simulink model "minseg_M2V3_2017a"  (R2017a)
settings: Solver=FixedStepDiscrete  StartTime=0.0  StopTime=inf  FixedStep=mdl_T_sample  RelTol=1e-3
undefined symbols (not defined in the file or in its folder): ctrl_lqr_K2, ctrl_motorDriver_v_ff_cmd_v_val, ctrl_motorDriver_v_ff_cmd_v_val_norm_dx_max, ctrl_motorDriver_v_ff_cmd_v_val_norm_dx_min, ctrl_motorDriver_v_output_max, ctrl_motorDriver_v_output_min, ctrl_motorDriver_v_pid_cmd_thetaDot_val, ctrl_motorDriver_v_pid_cmd_thetaDot_val_norm_dx_max, ctrl_motorDriver_v_pid_cmd_thetaDot_val_norm_dx_min, ctrl_motorDriver_v_pid_int_maxVal, ctrl_motorDriver_v_pid_int_minVal, ctrl_motorDriver_v_pid_k_d, ctrl_motorDriver_v_pid_k_i, ctrl_motorDriver_v_pid_k_p, ctrl_motorDriver_v_rts_ss_k_A, ctrl_motorDriver_v_rts_ss_k_B, ctrl_motorDriver_v_rts_ss_k_C, ctrl_motorDriver_v_rts_ss_k_D, ctrl_motorDriver_v_rts_ss_stateIC, ctrl_motorDriver_v_sfr_cmd_p_x_f, ctrl_motorDriver_v_sfr_cmd_p_x_mag, ctrl_motorDriver_v_sfr_cmd_p_y_f, ctrl_motorDriver_v_sfr_cmd_p_y_mag, ctrl_motorDriver_v_sfr_K, ctrl_motorDriver_v_sfr_K_plant, ctrl_motorDriver_v_sfr_K_rts, ctrl_motorDriver_v_T_cmd, ctrl_motorDriver_v_T_init, DiscIntNeverNeededParam, gyro_bias, io_srl_read_rateTransition_initialCondition, k_intmax_uint8, mdl_T_sample, mtr_encoder_filter_z_ss_A, mtr_encoder_filter_z_ss_B, mtr_encoder_filter_z_ss_C, mtr_encoder_filter_z_ss_D, plant, plant_accel_k_digital2analog, plant_body_l_c, plant_body_l_w, plant_gyro_encoder_filter_z_den, plant_gyro_encoder_filter_z_num, plant_gyro_filter_z_den, plant_gyro_filter_z_num, plant_gyro_k_digital2analog, plant_linear_ss_stateIC, plant_linear_ss_t_A, plant_linear_ss_t_B, plant_linear_ss_t_C, plant_linear_ss_t_D, plant_mtr_encoder_count2wheelRad, plant_mtr_encoder_filter_z_den, plant_mtr_encoder_filter_z_num, plant_pSupply_v, plant_supply_v, plant_T_init, plant_wheel_r
undefined symbols (not defined in the file): ctrl_lqr_addlDyn_A_discrete, ctrl_lqr_addlDyn_B_discrete, ctrl_lqr_addlDyn_C_discrete, ctrl_lqr_addlDyn_D_discrete, ctrl_lqr_addlDyn_k_antiWindup, ctrl_lqr_addlDyn_stateIC, plant_gyro_bias_movingAverage_n_pts, plant_linear_A_continuous, plant_linear_B_continuous, plant_linear_C_continuous, plant_linear_D_continuous, plant_linear_stateIC
libraries: svdutilitieslib x135, simulink x57, arduinolib x15, MinSegLibrary_M2V3 x3, dspindex x3, RASPlib x2
(part 6 of 6)

== system minseg_M2V3_2017a/Plant/Hardware/Calculations/Linear Position (p)/Wheel/Middle-Connected ==
  p.center.x : Inport
  p.center.y : Inport  Port=2
  p.center.z : Inport  Port=3
  body.angularPosition.y (yaw) : Inport  Port=4
  Add1 : Sum
  Add2 : Sum
  Bus Creator : BusCreator  Inputs=2
  Bus Creator1 : BusCreator  Inputs=2
  Bus Creator2 : BusCreator  Inputs=2
  Discrete Derivative [Average] : simulink/Discrete/Discrete Derivative  gainval=1.0  ICPrevScaledInput=0  OutMin=[]  OutMax=[]  OutDataType=fixdt(1, 16)  OutScaling=2^-10  DoSatur=off
      settings: AttributesFormatString=initialCondition = %<ICPrevScaledInput>
  Discrete Derivative [Left-Connected] : simulink/Discrete/Discrete Derivative  gainval=1.0  ICPrevScaledInput=0  OutMin=[]  OutMax=[]  OutDataType=fixdt(1, 16)  OutScaling=2^-10  DoSatur=off
      settings: AttributesFormatString=initialCondition = %<ICPrevScaledInput>
  Discrete Derivative [Middle-Connected] : simulink/Discrete/Discrete Derivative  gainval=1.0  ICPrevScaledInput=0  OutMin=[]  OutMax=[]  OutDataType=fixdt(1, 16)  OutScaling=2^-10  DoSatur=off
      settings: AttributesFormatString=initialCondition = %<ICPrevScaledInput>
  Gain3 : Gain  Gain=+ plant_body_l_w / 2
      settings: AttributesFormatString=%<Gain>
  Gain4 : Gain  Gain=- plant_body_l_w / 2
      settings: AttributesFormatString=%<Gain>
  Trigonometric Function : Trigonometry
  Trigonometric Function1 : Trigonometry  Operator=cos
  x : Outport
  y : Outport  Port=2
  z : Outport  Port=3
  wires:
  Discrete Derivative [Average]/1 -> Bus Creator2/2  "velocity [m/s]"
  Discrete Derivative [Middle-Connected]/1 -> Bus Creator1/2  "velocity [m/s]"
  Discrete Derivative [Left-Connected]/1 -> Bus Creator/2  "velocity [m/s]"
  Bus Creator1/1 -> y/1
  Bus Creator/1 -> x/1
  p.center.z/1 -> Bus Creator2/1, Discrete Derivative [Average]/1  "position [m]"
  Bus Creator2/1 -> z/1
  Add2/1 -> Discrete Derivative [Middle-Connected]/1, Bus Creator1/1  "position [m]"
  Add1/1 -> Bus Creator/1, Discrete Derivative [Left-Connected]/1  "position [m]"
  [yaw] -> Trigonometric Function/1
  Trigonometric Function/1 -> Gain3/1
  p.center.x/1 -> Add1/1
  Trigonometric Function1/1 -> Gain4/1
  p.center.y/1 -> Add2/1
  body.angularPosition.y (yaw)/1 -> [yaw]
  [yaw] -> Trigonometric Function1/1
  Gain3/1 -> Add1/2
  Gain4/1 -> Add2/2

== system minseg_M2V3_2017a/Plant/Hardware/Digital to Analog Conversion/Gyroscope/x/Moving Average ==
  u : Inport
  Enable : EnablePort
  Gain : Gain  Gain=ones(1,N) / N  Multiplication=Matrix(K*u)
      settings: AttributesFormatString=%<Gain>
  Mux : Mux  Inputs=2
  Unit Delay : UnitDelay  InitialCondition=zeros(N-1,1)  SampleTime=-1
  Variable Selector : dspindex/Variable Selector  NumInputs=1  rowsOrCols=Rows  IdxMode=Fixed  Elements=[ 1 : (N-1) ]  ZerOneIdxMode=One-based  errmode=Clip Index  FillMode=on  FillValues=0
  u.avg : Outport
  wires:
  Mux/1 -> Variable Selector/1, Gain/1
  Variable Selector/1 -> Unit Delay/1
  Gain/1 -> u.avg/1
  Unit Delay/1 -> Mux/2
  u/1 -> Mux/1

== system minseg_M2V3_2017a/Plant/Hardware/Digital to Analog Conversion/Gyroscope/y/Moving Average ==
  u : Inport
  Enable : EnablePort
  Gain : Gain  Gain=ones(1,N) / N  Multiplication=Matrix(K*u)
      settings: AttributesFormatString=%<Gain>
  Mux : Mux  Inputs=2
  Unit Delay : UnitDelay  InitialCondition=zeros(N-1,1)  SampleTime=-1
  Variable Selector : dspindex/Variable Selector  NumInputs=1  rowsOrCols=Rows  IdxMode=Fixed  Elements=[ 1 : (N-1) ]  ZerOneIdxMode=One-based  errmode=Clip Index  FillMode=on  FillValues=0
  u.avg : Outport
  wires:
  Mux/1 -> Variable Selector/1, Gain/1
  Variable Selector/1 -> Unit Delay/1
  Gain/1 -> u.avg/1
  Unit Delay/1 -> Mux/2
  u/1 -> Mux/1

== system minseg_M2V3_2017a/Plant/Hardware/Digital to Analog Conversion/Gyroscope/z/Moving Average ==
  u : Inport
  Enable : EnablePort
  Gain : Gain  Gain=ones(1,N) / N  Multiplication=Matrix(K*u)
      settings: AttributesFormatString=%<Gain>
  Mux : Mux  Inputs=2
  Unit Delay : UnitDelay  InitialCondition=zeros(N-1,1)  SampleTime=-1
  Variable Selector : dspindex/Variable Selector  NumInputs=1  rowsOrCols=Rows  IdxMode=Fixed  Elements=[ 1 : (N-1) ]  ZerOneIdxMode=One-based  errmode=Clip Index  FillMode=on  FillValues=0
  u.avg : Outport
  wires:
  Mux/1 -> Variable Selector/1, Gain/1
  Variable Selector/1 -> Unit Delay/1
  Gain/1 -> u.avg/1
  Unit Delay/1 -> Mux/2
  u/1 -> Mux/1

== system minseg_M2V3_2017a/Plant/Hardware-Equivalent Linear Dynamics/Calculation/Linear Position (p)/Wheel/Center ==
  wheel.angularVelocity.global : Inport
  body.angularPosition.y (yaw) : Inport  Port=2
  Add1 : Sum
  Bus Creator : BusCreator  Inputs=2
  Bus Creator1 : BusCreator  Inputs=2
  Bus Creator2 : BusCreator  Inputs=2
  Constant : Constant  Value=0  SampleTime=mdl_T_sample
  Constant1 : Constant  Value=plant.wheel.r  SampleTime=mdl_T_sample
      settings: AttributesFormatString=%<Value>
  Discrete-Time Integrator (X) : DiscreteIntegrator  InitialConditionSetting=State (most efficient)  SampleTime=-1  ICPrevOutput=DiscIntNeverNeededParam  ICPrevScaledInput=DiscIntNeverNeededParam
      settings: AttributesFormatString=initialCondition = %<InitialCondition>
  Discrete-Time Integrator (Y) : DiscreteIntegrator  InitialConditionSetting=State (most efficient)  SampleTime=-1  ICPrevOutput=DiscIntNeverNeededParam  ICPrevScaledInput=DiscIntNeverNeededParam
      settings: AttributesFormatString=initialCondition = %<InitialCondition>
  Discrete-Time Integrator (Z) : DiscreteIntegrator  InitialConditionSetting=State (most efficient)  SampleTime=-1  ICPrevOutput=DiscIntNeverNeededParam  ICPrevScaledInput=DiscIntNeverNeededParam
      settings: AttributesFormatString=initialCondition = %<InitialCondition>
  Gain3 : Gain  Gain=plant_wheel_r
      settings: AttributesFormatString=%<Gain>
  Gain4 : Gain  Gain=plant_wheel_r
      settings: AttributesFormatString=%<Gain>
  Product : Product
  Product1 : Product
  Trigonometric Function : Trigonometry  Operator=cos
  Trigonometric Function1 : Trigonometry
  x : Outport
  y : Outport  Port=2
  z : Outport  Port=3
  wires:
  Bus Creator2/1 -> z/1
  Bus Creator/1 -> x/1
  Bus Creator1/1 -> y/1
  Product/1 -> Discrete-Time Integrator (X)/1, Bus Creator/2  "velocity [m/s]"
  Product1/1 -> Discrete-Time Integrator (Y)/1, Bus Creator1/2  "velocity  [m/s]"
  Constant/1 -> Discrete-Time Integrator (Z)/1, Bus Creator2/2  "velocity [m/s]"
  Discrete-Time Integrator (X)/1 -> Bus Creator/1  "position [m]"
  Discrete-Time Integrator (Y)/1 -> Bus Creator1/1  "position [m]"
  Add1/1 -> Bus Creator2/1  "position [m]"
  wheel.angularVelocity.global/1 -> [theta_dot]
  Gain3/1 -> Product/1
  Trigonometric Function/1 -> Product/2
  body.angularPosition.y (yaw)/1 -> [yaw]
  Trigonometric Function1/1 -> Product1/2
  Gain4/1 -> Product1/1
  [yaw] -> Trigonometric Function/1
  [theta_dot] -> Gain3/1
  [theta_dot] -> Gain4/1
  [yaw] -> Trigonometric Function1/1
  Discrete-Time Integrator (Z)/1 -> Add1/2
  Constant1/1 -> Add1/1

== system minseg_M2V3_2017a/Plant/Hardware-Equivalent Linear Dynamics/Calculation/Linear Position (p)/Wheel/Left-Connected ==
  p.center.x : Inport
  p.center.y : Inport  Port=2
  p.center.z : Inport  Port=3
  body.angularPosition.y (yaw) : Inport  Port=4
  Add1 : Sum
  Add2 : Sum
  Bus Creator : BusCreator  Inputs=2
  Bus Creator1 : BusCreator  Inputs=2
  Bus Creator2 : BusCreator  Inputs=2
  Discrete Derivative (X) : simulink/Discrete/Discrete Derivative  gainval=1.0  ICPrevScaledInput=0  OutMin=[]  OutMax=[]  OutDataType=fixdt(1, 16)  OutScaling=2^-10  DoSatur=off
      settings: AttributesFormatString=initialCondition = %<ICPrevScaledInput>
  Discrete Derivative (Y) : simulink/Discrete/Discrete Derivative  gainval=1.0  ICPrevScaledInput=0  OutMin=[]  OutMax=[]  OutDataType=fixdt(1, 16)  OutScaling=2^-10  DoSatur=off
      settings: AttributesFormatString=initialCondition = %<ICPrevScaledInput>
  Discrete Derivative (Z) : simulink/Discrete/Discrete Derivative  gainval=1.0  ICPrevScaledInput=0  OutMin=[]  OutMax=[]  OutDataType=fixdt(1, 16)  OutScaling=2^-10  DoSatur=off
      settings: AttributesFormatString=initialCondition = %<ICPrevScaledInput>
  Gain3 : Gain  Gain=- plant_body_l_w / 2
      settings: AttributesFormatString=%<Gain>
  Gain4 : Gain  Gain=+ plant_body_l_w / 2
      settings: AttributesFormatString=%<Gain>
  Trigonometric Function : Trigonometry
  Trigonometric Function1 : Trigonometry  Operator=cos
  x : Outport
  y : Outport  Port=2
  z : Outport  Port=3
  wires:
  Gain4/1 -> Add2/2
  Gain3/1 -> Add1/2
  [yaw] -> Trigonometric Function1/1
  body.angularPosition.y (yaw)/1 -> [yaw]
  p.center.y/1 -> Add2/1
  Trigonometric Function1/1 -> Gain4/1
  p.center.x/1 -> Add1/1
  Trigonometric Function/1 -> Gain3/1
  [yaw] -> Trigonometric Function/1
  Add1/1 -> Discrete Derivative (X)/1, Bus Creator/1  "position [m]"
  Add2/1 -> Discrete Derivative (Y)/1, Bus Creator1/1  "position [m]"
  Bus Creator2/1 -> z/1
  p.center.z/1 -> Discrete Derivative (Z)/1, Bus Creator2/1  "position [m]"
  Bus Creator/1 -> x/1
  Bus Creator1/1 -> y/1
  Discrete Derivative (X)/1 -> Bus Creator/2  "velocity [m/s]"
  Discrete Derivative (Y)/1 -> Bus Creator1/2  "velocity [m/s]"
  Discrete Derivative (Z)/1 -> Bus Creator2/2  "velocity [m/s]"

== system minseg_M2V3_2017a/Plant/Hardware-Equivalent Linear Dynamics/Calculation/Linear Position (p)/Wheel/Middle-Connected ==
  p.center.x : Inport
  p.center.y : Inport  Port=2
  p.center.z : Inport  Port=3
  body.angularPosition.y (yaw) : Inport  Port=4
  Add1 : Sum
  Add2 : Sum
  Bus Creator : BusCreator  Inputs=2
  Bus Creator1 : BusCreator  Inputs=2
  Bus Creator2 : BusCreator  Inputs=2
  Discrete Derivative (X) : simulink/Discrete/Discrete Derivative  gainval=1.0  ICPrevScaledInput=0  OutMin=[]  OutMax=[]  OutDataType=fixdt(1, 16)  OutScaling=2^-10  DoSatur=off
      settings: AttributesFormatString=initialCondition = %<ICPrevScaledInput>
  Discrete Derivative (Y) : simulink/Discrete/Discrete Derivative  gainval=1.0  ICPrevScaledInput=0  OutMin=[]  OutMax=[]  OutDataType=fixdt(1, 16)  OutScaling=2^-10  DoSatur=off
      settings: AttributesFormatString=initialCondition = %<ICPrevScaledInput>
  Discrete Derivative (Z) : simulink/Discrete/Discrete Derivative  gainval=1.0  ICPrevScaledInput=0  OutMin=[]  OutMax=[]  OutDataType=fixdt(1, 16)  OutScaling=2^-10  DoSatur=off
      settings: AttributesFormatString=initialCondition = %<ICPrevScaledInput>
  Gain3 : Gain  Gain=+ plant_body_l_w / 2
      settings: AttributesFormatString=%<Gain>
  Gain4 : Gain  Gain=- plant_body_l_w / 2
      settings: AttributesFormatString=%<Gain>
  Trigonometric Function : Trigonometry
  Trigonometric Function1 : Trigonometry  Operator=cos
  x : Outport
  y : Outport  Port=2
  z : Outport  Port=3
  wires:
  Discrete Derivative (Z)/1 -> Bus Creator2/2  "velocity [m/s]"
  Discrete Derivative (Y)/1 -> Bus Creator1/2  "velocity [m/s]"
  Discrete Derivative (X)/1 -> Bus Creator/2  "velocity  [m/s]"
  Bus Creator1/1 -> y/1
  Bus Creator/1 -> x/1
  p.center.z/1 -> Discrete Derivative (Z)/1, Bus Creator2/1  "position [m]"
  Bus Creator2/1 -> z/1
  Add2/1 -> Discrete Derivative (Y)/1, Bus Creator1/1  "position [m]"
  Add1/1 -> Discrete Derivative (X)/1, Bus Creator/1  "position [m]"
  [yaw] -> Trigonometric Function/1
  Trigonometric Function/1 -> Gain3/1
  p.center.x/1 -> Add1/1
  Trigonometric Function1/1 -> Gain4/1
  p.center.y/1 -> Add2/1
  body.angularPosition.y (yaw)/1 -> [yaw]
  [yaw] -> Trigonometric Function1/1
  Gain3/1 -> Add1/2
  Gain4/1 -> Add2/2

== system minseg_M2V3_2017a/User IO/Reads (From PC)/Controller/State Feedback Regulation/[x,y] to [magnitude, angle]: p/Angle ==
  u.x : Inport
  u.y : Inport  Port=2
  Trigonometric Function : Trigonometry  Operator=atan2
  "< u  " : Outport
  wires:
  u.x/1 -> Trigonometric Function/2
  u.y/1 -> Trigonometric Function/1
  Trigonometric Function/1 -> "< u  "/1

== system minseg_M2V3_2017a/User IO/Reads (From PC)/Controller/State Feedback Regulation/[x,y] to [magnitude, angle]: p/Magnitude ==
  u.x : Inport
  u.y : Inport  Port=2
  Add : Sum
  Constant1 : Constant  Value=2  SampleTime=mdl_T_sample
  Constant2 : Constant  Value=2  SampleTime=mdl_T_sample
  Math Function : Math  Operator=pow  SaturateOnIntegerOverflow=on
  Math Function1 : Math  Operator=pow  SaturateOnIntegerOverflow=on
  Sqrt : Sqrt  SaturateOnIntegerOverflow=on
  | u | : Outport
  wires:
  Math Function1/1 -> Add/2
  u.x/1 -> Math Function/1
  Math Function/1 -> Add/1
  Constant2/1 -> Math Function/2
  Constant1/1 -> Math Function1/2
  Sqrt/1 -> | u |/1
  Add/1 -> Sqrt/1
  u.y/1 -> Math Function1/1

== system minseg_M2V3_2017a/User IO/Reads (From PC)/Controller/State Feedback Regulation/[x,y] to [magnitude, angle]: p.dot/Angle ==
  u.x : Inport
  u.y : Inport  Port=2
  Trigonometric Function : Trigonometry  Operator=atan2
  "< u  " : Outport
  wires:
  Trigonometric Function/1 -> "< u  "/1
  u.y/1 -> Trigonometric Function/1
  u.x/1 -> Trigonometric Function/2

== system minseg_M2V3_2017a/User IO/Reads (From PC)/Controller/State Feedback Regulation/[x,y] to [magnitude, angle]: p.dot/Magnitude ==
  u.x : Inport
  u.y : Inport  Port=2
  Add : Sum
  Constant1 : Constant  Value=2  SampleTime=mdl_T_sample
  Constant2 : Constant  Value=2  SampleTime=mdl_T_sample
  Math Function : Math  Operator=pow  SaturateOnIntegerOverflow=on
  Math Function1 : Math  Operator=pow  SaturateOnIntegerOverflow=on
  Sqrt : Sqrt  SaturateOnIntegerOverflow=on
  | u | : Outport
  wires:
  u.y/1 -> Math Function1/1
  Add/1 -> Sqrt/1
  Sqrt/1 -> | u |/1
  Constant1/1 -> Math Function1/2
  Constant2/1 -> Math Function/2
  Math Function/1 -> Add/1
  u.x/1 -> Math Function/1
  Math Function1/1 -> Add/2

== system minseg_M2V3_2017a/User IO/Writes (To PC)/Plant: Linear Dynamics/Controller: PID/Standard/Pass Through ==
  In1 : Inport
  In2 : Inport  Port=2
  In3 : Inport  Port=3
  In4 : Inport  Port=4
  Out1 : Outport
  Out2 : Outport  Port=2
  Out3 : Outport  Port=3
  Out4 : Outport  Port=4
  wires:
  In1/1 -> Out1/1
  In2/1 -> Out2/1
  In3/1 -> Out3/1
  In4/1 -> Out4/1

== system minseg_M2V3_2017a/User IO/Writes (To PC)/Plant: Linear Dynamics/Controller: PID/Standard/Wheel ==
  wheel.angularVelocity.global : Inport
  body.angularPosition.y (yaw) : Inport  Port=2
  Bus Creator : BusCreator  Inputs=3
  Bus Creator1 : BusCreator  Inputs=3
  Bus Creator2 : BusCreator  Inputs=3
  Bus Selector3 : BusSelector  OutputSignals=x.position [m],y.position [m],z.position [m]
  Bus Selector4 : BusSelector  OutputSignals=x.position [m],y.position [m],z.position [m]
  Center : Subsystem
  Left-Connected : Subsystem
  Middle-Connected : Subsystem
  left : Outport
  middle : Outport  Port=2
  center : Outport  Port=3
  wires:
  Bus Creator/1 -> left/1
  Bus Creator1/1 -> middle/1
  body.angularPosition.y (yaw)/1 -> [yaw]
  wheel.angularVelocity.global/1 -> Center/1(wheel.angularVelocity.global)
  Left-Connected/1(x) -> Bus Creator/1  "x"
  Left-Connected/2(y) -> Bus Creator/2  "y"
  Left-Connected/3(z) -> Bus Creator/3  "z"
  Middle-Connected/1(x) -> Bus Creator1/1  "x"
  Middle-Connected/2(y) -> Bus Creator1/2  "y"
  Middle-Connected/3(z) -> Bus Creator1/3  "z"
  Center/1(x) -> Bus Creator2/1  "x"
  Center/2(y) -> Bus Creator2/2  "y"
  Center/3(z) -> Bus Creator2/3  "z"
  Bus Creator2/1 -> [p_center], center/1
  [yaw] -> Center/2(body.angularPosition.y (yaw))
  [yaw] -> Middle-Connected/4(body.angularPosition.y (yaw))
  [p_center] -> Bus Selector3/1
  Bus Selector3/1 -> Middle-Connected/1(p.center.x)  "<position [m]>"
  Bus Selector3/2 -> Middle-Connected/2(p.center.y)  "<position [m]>"
  Bus Selector3/3 -> Middle-Connected/3(p.center.z)  "<position [m]>"
  Bus Selector4/3 -> Left-Connected/3(p.center.z)  "<position [m]>"
  Bus Selector4/2 -> Left-Connected/2(p.center.y)  "<position [m]>"
  Bus Selector4/1 -> Left-Connected/1(p.center.x)  "<position [m]>"
  [p_center] -> Bus Selector4/1
  [yaw] -> Left-Connected/4(body.angularPosition.y (yaw))

== system minseg_M2V3_2017a/Plant/Hardware/Calculations/Body Angular Position (phi)/Z (Roll)/Accelerometer/Derivative ==
  x : Inport
  Discrete Derivative : simulink/Discrete/Discrete Derivative  gainval=1.0  ICPrevScaledInput=0  OutMin=[]  OutMax=[]  OutDataType=fixdt(1, 16)  OutScaling=2^-10  DoSatur=off
      settings: AttributesFormatString=initialCondition = %<ICPrevScaledInput>
  Discrete Filter: Bessel LPF : DiscreteFilter  Numerator=plant_mtr_encoder_filter_z_num  Denominator=plant_mtr_encoder_filter_z_den  SampleTime=mdl_T_sample
      settings: AttributesFormatString=|
      | Num: %<Numerator>
      | Den: %<Denominator>
  State-Space: Bessel LPF : DiscreteStateSpace  Commented=through  A=mtr_encoder_filter_z_ss_A  B=mtr_encoder_filter_z_ss_B  C=mtr_encoder_filter_z_ss_C  D=mtr_encoder_filter_z_ss_D  X0=[0 0]  SampleTime=mdl_T_sample
      settings: AttributesFormatString=|
      | A: %<A>
      | B: %<B>
      | C: %<C>
      | D: %<D>
  x.dot : Outport
  wires:
  x/1 -> Discrete Derivative/1
  Discrete Derivative/1 -> State-Space: Bessel LPF/1
  Discrete Filter: Bessel LPF/1 -> x.dot/1
  State-Space: Bessel LPF/1 -> Discrete Filter: Bessel LPF/1

== system minseg_M2V3_2017a/User IO/Writes (To PC)/Plant: Linear Dynamics/Controller: PID/Standard/Wheel/Center ==
  wheel.angularVelocity.global : Inport
  body.angularPosition.y (yaw) : Inport  Port=2
  Add1 : Sum
  Bus Creator : BusCreator  Inputs=2
  Bus Creator1 : BusCreator  Inputs=2
  Bus Creator2 : BusCreator  Inputs=2
  Constant : Constant  Value=0  SampleTime=mdl_T_sample
  Constant1 : Constant  Value=plant.wheel.r  SampleTime=mdl_T_sample
      settings: AttributesFormatString=%<Value>
  Discrete-Time Integrator (X) : DiscreteIntegrator  InitialConditionSetting=State (most efficient)  SampleTime=-1  ICPrevOutput=DiscIntNeverNeededParam  ICPrevScaledInput=DiscIntNeverNeededParam
      settings: AttributesFormatString=initialCondition = %<InitialCondition>
  Discrete-Time Integrator (Y) : DiscreteIntegrator  InitialConditionSetting=State (most efficient)  SampleTime=-1  ICPrevOutput=DiscIntNeverNeededParam  ICPrevScaledInput=DiscIntNeverNeededParam
      settings: AttributesFormatString=initialCondition = %<InitialCondition>
  Discrete-Time Integrator (Z) : DiscreteIntegrator  InitialConditionSetting=State (most efficient)  SampleTime=-1  ICPrevOutput=DiscIntNeverNeededParam  ICPrevScaledInput=DiscIntNeverNeededParam
      settings: AttributesFormatString=initialCondition = %<InitialCondition>
  Gain3 : Gain  Gain=plant_wheel_r
      settings: AttributesFormatString=%<Gain>
  Gain4 : Gain  Gain=plant_wheel_r
      settings: AttributesFormatString=%<Gain>
  Product : Product
  Product1 : Product
  Trigonometric Function : Trigonometry  Operator=cos
  Trigonometric Function1 : Trigonometry
  x : Outport
  y : Outport  Port=2
  z : Outport  Port=3
  wires:
  Bus Creator2/1 -> z/1
  Bus Creator/1 -> x/1
  Bus Creator1/1 -> y/1
  Product/1 -> Discrete-Time Integrator (X)/1, Bus Creator/2  "velocity [m/s]"
  Product1/1 -> Discrete-Time Integrator (Y)/1, Bus Creator1/2  "velocity  [m/s]"
  Constant/1 -> Discrete-Time Integrator (Z)/1, Bus Creator2/2  "velocity [m/s]"
  Discrete-Time Integrator (X)/1 -> Bus Creator/1  "position [m]"
  Discrete-Time Integrator (Y)/1 -> Bus Creator1/1  "position [m]"
  Add1/1 -> Bus Creator2/1  "position [m]"
  wheel.angularVelocity.global/1 -> [theta_dot]
  Gain3/1 -> Product/1
  Trigonometric Function/1 -> Product/2
  body.angularPosition.y (yaw)/1 -> [yaw]
  Trigonometric Function1/1 -> Product1/2
  Gain4/1 -> Product1/1
  [yaw] -> Trigonometric Function/1
  [theta_dot] -> Gain3/1
  [theta_dot] -> Gain4/1
  [yaw] -> Trigonometric Function1/1
  Discrete-Time Integrator (Z)/1 -> Add1/2
  Constant1/1 -> Add1/1

== system minseg_M2V3_2017a/User IO/Writes (To PC)/Plant: Linear Dynamics/Controller: PID/Standard/Wheel/Left-Connected ==
  p.center.x : Inport
  p.center.y : Inport  Port=2
  p.center.z : Inport  Port=3
  body.angularPosition.y (yaw) : Inport  Port=4
  Add1 : Sum
  Add2 : Sum
  Bus Creator : BusCreator  Inputs=2
  Bus Creator1 : BusCreator  Inputs=2
  Bus Creator2 : BusCreator  Inputs=2
  Discrete Derivative (X) : simulink/Discrete/Discrete Derivative  gainval=1.0  ICPrevScaledInput=0  OutMin=[]  OutMax=[]  OutDataType=fixdt(1, 16)  OutScaling=2^-10  DoSatur=off
      settings: AttributesFormatString=initialCondition = %<ICPrevScaledInput>
  Discrete Derivative (Y) : simulink/Discrete/Discrete Derivative  gainval=1.0  ICPrevScaledInput=0  OutMin=[]  OutMax=[]  OutDataType=fixdt(1, 16)  OutScaling=2^-10  DoSatur=off
      settings: AttributesFormatString=initialCondition = %<ICPrevScaledInput>
  Discrete Derivative (Z) : simulink/Discrete/Discrete Derivative  gainval=1.0  ICPrevScaledInput=0  OutMin=[]  OutMax=[]  OutDataType=fixdt(1, 16)  OutScaling=2^-10  DoSatur=off
      settings: AttributesFormatString=initialCondition = %<ICPrevScaledInput>
  Gain3 : Gain  Gain=- plant_body_l_w / 2
      settings: AttributesFormatString=%<Gain>
  Gain4 : Gain  Gain=+ plant_body_l_w / 2
      settings: AttributesFormatString=%<Gain>
  Trigonometric Function : Trigonometry
  Trigonometric Function1 : Trigonometry  Operator=cos
  x : Outport
  y : Outport  Port=2
  z : Outport  Port=3
  wires:
  Gain4/1 -> Add2/2
  Gain3/1 -> Add1/2
  [yaw] -> Trigonometric Function1/1
  body.angularPosition.y (yaw)/1 -> [yaw]
  p.center.y/1 -> Add2/1
  Trigonometric Function1/1 -> Gain4/1
  p.center.x/1 -> Add1/1
  Trigonometric Function/1 -> Gain3/1
  [yaw] -> Trigonometric Function/1
  Add1/1 -> Discrete Derivative (X)/1, Bus Creator/1  "position [m]"
  Add2/1 -> Discrete Derivative (Y)/1, Bus Creator1/1  "position [m]"
  Bus Creator2/1 -> z/1
  p.center.z/1 -> Discrete Derivative (Z)/1, Bus Creator2/1  "position [m]"
  Bus Creator/1 -> x/1
  Bus Creator1/1 -> y/1
  Discrete Derivative (X)/1 -> Bus Creator/2  "velocity [m/s]"
  Discrete Derivative (Y)/1 -> Bus Creator1/2  "velocity [m/s]"
  Discrete Derivative (Z)/1 -> Bus Creator2/2  "velocity [m/s]"

== system minseg_M2V3_2017a/User IO/Writes (To PC)/Plant: Linear Dynamics/Controller: PID/Standard/Wheel/Middle-Connected ==
  p.center.x : Inport
  p.center.y : Inport  Port=2
  p.center.z : Inport  Port=3
  body.angularPosition.y (yaw) : Inport  Port=4
  Add1 : Sum
  Add2 : Sum
  Bus Creator : BusCreator  Inputs=2
  Bus Creator1 : BusCreator  Inputs=2
  Bus Creator2 : BusCreator  Inputs=2
  Discrete Derivative (X) : simulink/Discrete/Discrete Derivative  gainval=1.0  ICPrevScaledInput=0  OutMin=[]  OutMax=[]  OutDataType=fixdt(1, 16)  OutScaling=2^-10  DoSatur=off
      settings: AttributesFormatString=initialCondition = %<ICPrevScaledInput>
  Discrete Derivative (Y) : simulink/Discrete/Discrete Derivative  gainval=1.0  ICPrevScaledInput=0  OutMin=[]  OutMax=[]  OutDataType=fixdt(1, 16)  OutScaling=2^-10  DoSatur=off
      settings: AttributesFormatString=initialCondition = %<ICPrevScaledInput>
  Discrete Derivative (Z) : simulink/Discrete/Discrete Derivative  gainval=1.0  ICPrevScaledInput=0  OutMin=[]  OutMax=[]  OutDataType=fixdt(1, 16)  OutScaling=2^-10  DoSatur=off
      settings: AttributesFormatString=initialCondition = %<ICPrevScaledInput>
  Gain3 : Gain  Gain=+ plant_body_l_w / 2
      settings: AttributesFormatString=%<Gain>
  Gain4 : Gain  Gain=- plant_body_l_w / 2
      settings: AttributesFormatString=%<Gain>
  Trigonometric Function : Trigonometry
  Trigonometric Function1 : Trigonometry  Operator=cos
  x : Outport
  y : Outport  Port=2
  z : Outport  Port=3
  wires:
  Discrete Derivative (Z)/1 -> Bus Creator2/2  "velocity [m/s]"
  Discrete Derivative (Y)/1 -> Bus Creator1/2  "velocity [m/s]"
  Discrete Derivative (X)/1 -> Bus Creator/2  "velocity  [m/s]"
  Bus Creator1/1 -> y/1
  Bus Creator/1 -> x/1
  p.center.z/1 -> Discrete Derivative (Z)/1, Bus Creator2/1  "position [m]"
  Bus Creator2/1 -> z/1
  Add2/1 -> Discrete Derivative (Y)/1, Bus Creator1/1  "position [m]"
  Add1/1 -> Discrete Derivative (X)/1, Bus Creator/1  "position [m]"
  [yaw] -> Trigonometric Function/1
  Trigonometric Function/1 -> Gain3/1
  p.center.x/1 -> Add1/1
  Trigonometric Function1/1 -> Gain4/1
  p.center.y/1 -> Add2/1
  body.angularPosition.y (yaw)/1 -> [yaw]
  [yaw] -> Trigonometric Function1/1
  Gain3/1 -> Add1/2
  Gain4/1 -> Add2/2
